simulink model "G24i_buck_boost"  (R2014a)
settings: Solver=ode23tb  StartTime=0.0  StopTime=5  RelTol=1e-4
values from neighbouring files (symbols this model uses):
  Array_Voc = [0.328644000009 2.76811 3.09396940822 3.26133568944 3.36629977409 3.44398192097 3.50365713438 3.55225637345 3.59363766529 3.63021764721 3.6624 3.69037314882 ... (101 elements, 101x1)]    [Array_Voc.mat]
  ArrayCurrent = [1.05303e-05 0.0329007487024 0.0659314357778 0.100205 0.132978217474 0.166891516648 0.200872978445 0.234107600227 0.267513340222 0.302009988541 0.336322 0.36979130469 ... (44440 elements, 101x440)]    [ArrayCurrent.mat]    (also in Genrate_SC_mod.m = fitresult_normal_g42(V,G); temp3.m = fitresult(V,G))
  ArrayVoltage = [0 0.01 0.02 0.03 0.04 0.05 0.06 0.07 0.08 0.09 0.1 0.11 ... (440 elements, 1x440)]    [ArrayVoltage.mat]    (also in Genrate_SC_mod.m = (0:0.01:max(Voltage)); temp3.m = (0:0.01:max(Voltage)))
  Irradiance = (min(Lux):50:max(Lux))    [Genrate_SC_mod.m]    (also in Irradiance.mat = [0 50 100 150 200 250 300 350 400 450 500 550 ... (101 eleme; temp3.m)
undefined symbols (not defined in the file or in its folder): sigbuilder_block
libraries: powerlib x16, simulink_extras x3, simulink x1
settings Model: NumberOfSteps=5  Creator=kartik.karuna  LastModifiedBy=kartik.karuna
settings SolverCC: SolverJacobianMethodControl=SparseAnalytical  ZeroCrossAlgorithm=Adaptive

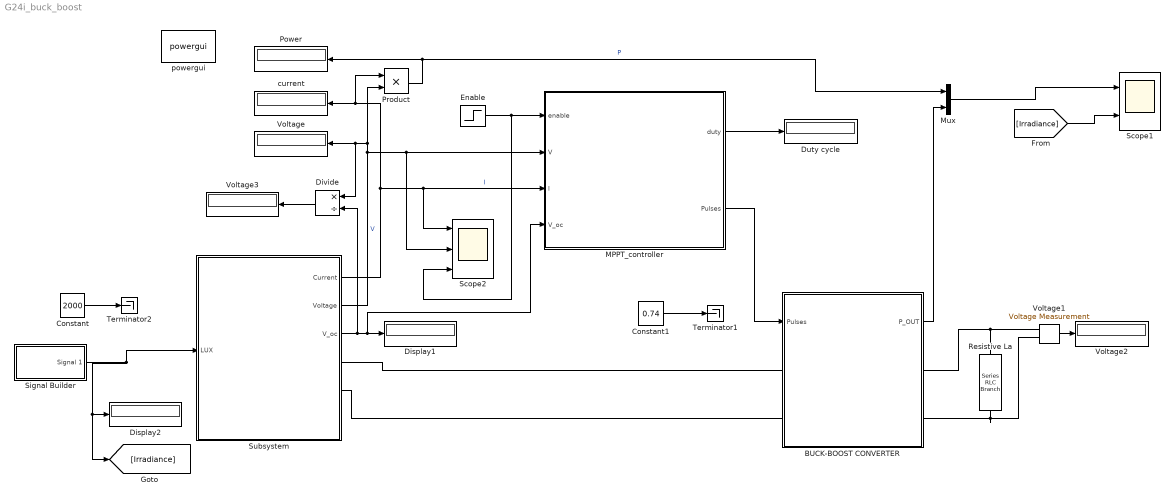
== system G24i_buck_boost ==
  BUCK-BOOST CONVERTER : Subsystem
  Constant : Constant  Value=2000
  Constant1 : Constant  Value=0.74
  Display1 : Display
  Display2 : Display
  Divide : Product  Inputs=*/
  Duty cycle : Display
  Enable : Step  Time=0.02  SampleTime=0
  MPPT_controller : Subsystem  Variant=on
  Mux : Mux  Inputs=2
  Power : Display
  Product : Product  RndMeth=Zero
  Resistive La : powerlib/Elements/Series RLC Branch  LConnTagsString=__new0  RConnTagsString=__new0  BranchType=R  Resistance=30  Inductance=1e-3  SetiL0=off  InitialCurrent=0  Capacitance=1e-6  Setx0=off  InitialVoltage=0  Measurements=None
  Scope1 : Scope  NumInputPorts=2
      settings: TimeRange=0.5  YMin=0~300  YMax=5.75~2500  SaveName=ScopeData2
  Scope2 : Scope  NumInputPorts=3
      settings: TimeRange=0.09  YMin=0.3125~3.9575~0.95  YMax=0.3475~3.968~1.05
  Signal Builder : Subsystem  Tag=STV Subsys  LoadFcn=sigbuilder_block('load');  StartFcn=sigbuilder_block('start');  StopFcn=sigbuilder_block('stop');  ClipboardFcn=sigbuilder_block('clipboard');  mask(Sigbuilder block){}
      mask help: Simulink:masks:SigbuilderBlock_MD
      mask init:
      | if ~strcmp(get_param(bdroot(gcbh),'SimulationStatus'),'stopped') tuvar = sigbuilder_block('maskInit'); end
      settings: CopyFcn=sigbuilder_block('copy');  DeleteFcn=sigbuilder_block('delete');  ModelCloseFcn=sigbuilder_block('modelClose');  PreSaveFcn=sigbuilder_block('preSave');  PauseFcn=sigbuilder_block('pause');  ContinueFcn=sigbuilder_block('continue');  NameChangeFcn=sigbuilder_block('namechange');  OpenFcn=sigbuilder_block('open',[310.966 125.379 1271.79 657.31 ]);  CloseFcn=sigbuilder_block('close');
      mask Display: plot(0, 0, 100, 100,[2, 2, 32, 32, 2], [68, 8, 8, 68, 68],[32, 2], [38, 38], [32, 19, 2],[53, 60, 44], [32, 17, 17, 2],[16, 16, 31, 31]);txt = getActiveGroup(gcbh);text(2, 100, txt,'verticalAlignment', 'top');
  Subsystem : Subsystem
  Terminator1 : Terminator
  Terminator2 : Terminator
  Voltage : Display
  Voltage1 : powerlib/Measurements/Voltage Measurement  PhasorSimulation=off  OutputType=Complex  PSBequivalent=0
  Voltage2 : Display
  Voltage3 : Display
  current : Display
  powergui : powerlib/powergui  Priority=1  SimulationMode=Continuous  SolverType=Tustin  SampleTime=50e-6  frequency=50  SPID=off  DisableSnubberDevices=off  DisableRonSwitches=off  DisableVfSwitches=off  SwTol=0  Interpol=off  DisplayEquations=off  Ts=0  methode=off  frequencyindice=0  Pbase=100e6  ErrMax=1e-4  Iterations=50  UnitsV=kV  UnitsW=MW  FunctionMessages=off  echomessages=off  HookPort=off  EnableUseOfTLC=off  x0status=blocks  RestoreLinks=warning  ResistiveCurrentMeasurement=off  Frange=[0:2:500]  Ylog=off  Xlog=on  ShowGrid=off  save=off  variable=ZData  structure=0  ZoomFFT=off  StartTime=0.0  cycles=1  DisplayStyle=1  fundamental=60  FreqAxis=off  MaxFrequency=1000  frequencyindicesteady=1  RmsSteady=1  display=off
  wires:
  BUCK-BOOST CONVERTER/1(P_OUT) -> Mux/2
  Mux/1 -> Scope1/1
  Product/1 -> Power/1, Mux/1  "P"
  Voltage1/1 -> Voltage2/1
  Enable/1 -> MPPT_controller/1(enable), Scope2/3
  Subsystem/3("V_oc ") -> Divide/2, MPPT_controller/4(V_oc), Display1/1
  Divide/1 -> Voltage3/1
  MPPT_controller/1(duty) -> Duty cycle/1
  Signal Builder/1(Signal 1) -> [Irradiance], Display2/1, Subsystem/1(LUX)
  Subsystem/2(Voltage) -> Product/2, Divide/1, Voltage/1, MPPT_controller/2(V), Scope2/2  "V"
  Subsystem/1(Current) -> Product/1, current/1, MPPT_controller/3(I), Scope2/1  "I"
  MPPT_controller/2(Pulses) -> BUCK-BOOST CONVERTER/1(Pulses)
  Constant1/1 -> Terminator1/1
  Constant/1 -> Terminator2/1
  [Irradiance] -> Scope1/2
  connections:
  Resistive La/RConn1 -- Voltage1/LConn2 -- BUCK-BOOST CONVERTER/RConn2
  Resistive La/LConn1 -- Voltage1/LConn1 -- BUCK-BOOST CONVERTER/RConn1
  BUCK-BOOST CONVERTER/LConn1 -- Subsystem/RConn1
  BUCK-BOOST CONVERTER/LConn2 -- Subsystem/RConn2

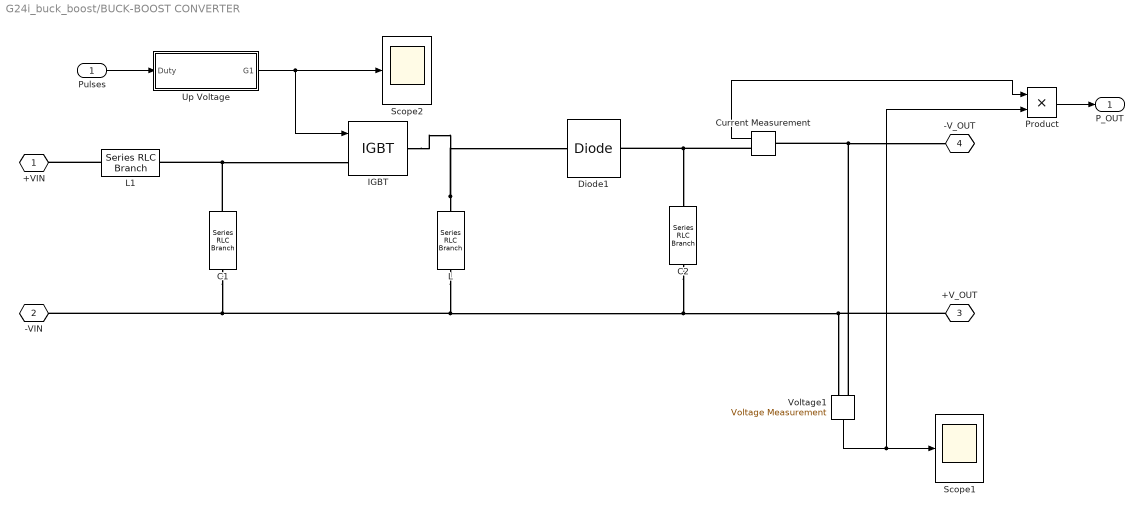
== system G24i_buck_boost/BUCK-BOOST CONVERTER ==
  Pulses : Inport
  " C1" : powerlib/Elements/Series RLC Branch  LConnTagsString=__new0  RConnTagsString=__new0  BranchType=C  Resistance=5  Inductance=0.05  SetiL0=off  InitialCurrent=0  Capacitance=2000e-6  Setx0=on  InitialVoltage=0  Measurements=Branch voltage and current
  " C2" : powerlib/Elements/Series RLC Branch  LConnTagsString=__new0  RConnTagsString=__new0  BranchType=C  Resistance=5  Inductance=0.05  SetiL0=off  InitialCurrent=0  Capacitance=2000e-6  Setx0=on  InitialVoltage=0  Measurements=Branch voltage and current
  " L" : powerlib/Elements/Series RLC Branch  LConnTagsString=__new0  RConnTagsString=__new0  BranchType=L  Resistance=5  Inductance=47e-6  SetiL0=on  InitialCurrent=0  Capacitance=1.0  Setx0=off  InitialVoltage=0  Measurements=Branch voltage and current
  " L1" : powerlib/Elements/Series RLC Branch  LConnTagsString=__new0  RConnTagsString=__new0  BranchType=L  Resistance=5  Inductance=1000e-6  SetiL0=on  InitialCurrent=0  Capacitance=1.0  Setx0=off  InitialVoltage=0  Measurements=Branch voltage and current
  Current Measurement : powerlib/Measurements/Current Measurement  PhasorSimulation=off  OutputType=Complex  PSBequivalent=0
  Diode1 : powerlib/Power Electronics/Diode  Ron=0.00001  Lon=0  Vf=0.8  IC=0  UseSnubber=off  Rs=1e4  Cs=1e-4  Measurements=off
  IGBT : powerlib/Power Electronics/IGBT  Ron=0.00001  Lon=0  Vf=2.5  Tf=1e-6  Tt=1e4  IC=0  Rs=1e5  Cs=inf  Measurements=off
  Product : Product  RndMeth=Zero
  Scope1 : Scope
      settings: TimeRange=1  YMin=1.478  YMax=1.497
  Scope2 : Scope
      settings: TimeRange=1  YMin=1.478  YMax=1.497  SaveName=ScopeData3
  Up Voltage : Subsystem  mask{fc=10000, Gama=0.5}
      mask prompts: fc "Frequency (Hz)"; Gama "Duty Cycle  (0-1)"
      mask Display: disp('CONTROL SIGNAL')
  Voltage1 : powerlib/Measurements/Voltage Measurement  PhasorSimulation=off  OutputType=Complex  PSBequivalent=0
  +VIN : PMIOPort  Tag=PMCPort  Port=1  Side=Left
  -VIN : PMIOPort  Tag=PMCPort  Port=2  Side=Left
  +V_OUT : PMIOPort  Tag=PMCPort  Port=3  Side=Right
  -V_OUT : PMIOPort  Tag=PMCPort  Port=4  Side=Right
  P_OUT : Outport
  wires:
  Voltage1/1 -> Scope1/1, Product/2
  Pulses/1 -> Up Voltage/1(Duty)
  Up Voltage/1(G1) -> IGBT/1, Scope2/1
  Current Measurement/1 -> Product/1
  Product/1 -> P_OUT/1
  connections:
  Voltage1/LConn2 -- -V_OUT/RConn1 -- Current Measurement/LConn1
  " L"/RConn1 -- +V_OUT/RConn1 -- Voltage1/LConn1 -- " C2"/RConn1 -- " C1"/RConn1 -- -VIN/RConn1
  " L"/LConn1 -- IGBT/RConn1 -- Diode1/RConn1
  " C1"/LConn1 -- IGBT/LConn1 -- " L1"/LConn1
  Current Measurement/RConn1 -- Diode1/LConn1 -- " C2"/LConn1
  " L1"/RConn1 -- +VIN/RConn1

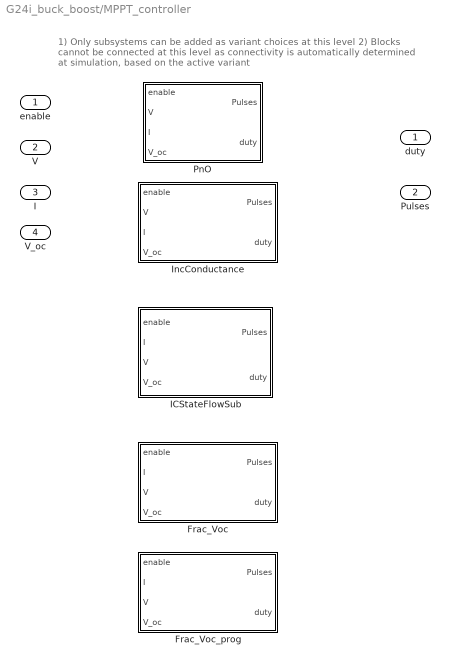
== system G24i_buck_boost/MPPT_controller ==
  note: 1) Only subsystems can be added as variant choices at this level
      | 2) Blocks cannot be connected at this level as connectivity is
      | automatically determined at simulation, based on the active variant
  enable : Inport
  V : Inport  Port=2
  I : Inport  Port=3
  V_oc : Inport  Port=4
  Frac_Voc : Subsystem  VariantControl=MPPT_Frac_Voc
  Frac_Voc_prog : Subsystem  VariantControl=MPPT_Frac_Voc_prog
  ICStateFlowSub : Subsystem  VariantControl=MPPT_IC_SF
  IncConductance : Subsystem  VariantControl=MPPT_IC_logic
  PnO : Subsystem  VariantControl=MPPT_PnO
  duty : Outport
  Pulses : Outport  Port=2

== system G24i_buck_boost/Signal Builder ==
  Demux : Demux  Tag=STV Demux  Outputs=1
  FromWs : FromWorkspace  Tag=STV FromWs  VariableName=tuvar  SampleTime=0
      SigBuilderData=|
      | common.afterFinalStr = 'Extrapolate'
      | common.sampleTime = 0
      | dataSet.timeRange = [0 2]
      | dataSet.name = 'Group 1'
      | sbobj.Groups.Name = 'Group 1'
      | sbobj.Groups.Signals.Name = 'Signal 1'
      | sbobj.Groups.Signals.XData = [0 0.35 0.55 0.85 1.2 2]
      | sbobj.Groups.Signals.YData = [2500 2500 200 200 800 800]
      | sbobj.Groups.TimeRange = [0 2]
  Signal 1 : Outport  Tag=STV Outport
  wires:
  Demux/1 -> Signal 1/1
  FromWs/1 -> Demux/1

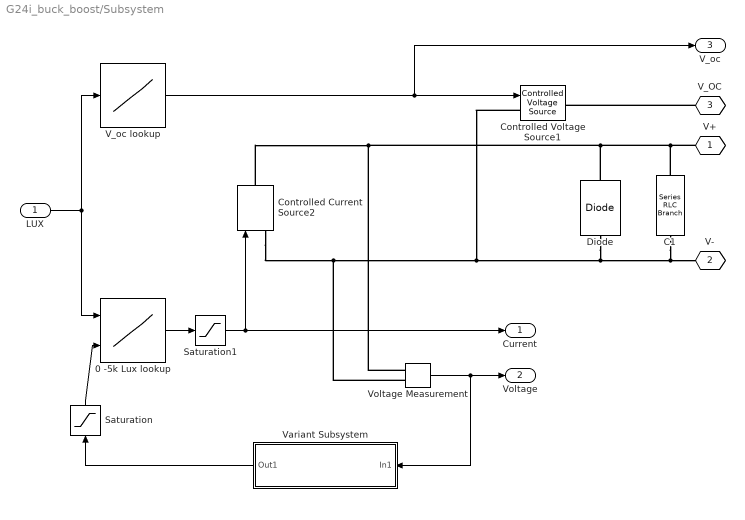
== system G24i_buck_boost/Subsystem ==
  LUX : Inport
  " C1" : powerlib/Elements/Series RLC Branch  LConnTagsString=__new0  RConnTagsString=__new0  BranchType=C  Resistance=5  Inductance=0.05  SetiL0=off  InitialCurrent=0  Capacitance=100e-6  Setx0=on  InitialVoltage=0  Measurements=Branch voltage and current
  0 -5k Lux lookup : Lookup_n-D  BreakpointsForDimension1=Irradiance  BreakpointsForDimension2=ArrayVoltage  BreakpointsForDimension1Min=[0]  BreakpointsForDimension2Min=[0]  BreakpointsForDimension1Max=[5000]  BreakpointsForDimension2Max=[6]  Table=ArrayCurrent  DiagnosticForOutOfRangeInput=Warning  RndMeth=Simplest  InputSameDT=on
  Controlled Current Source2 : powerlib/Electrical Sources/Controlled Current Source  Initialize=on  Source_Type=DC  Amplitude=0  Phase=0  Frequency=0  Measurements=None
  Controlled Voltage Source1 : powerlib/Electrical Sources/Controlled Voltage Source  Initialize=on  Source_Type=AC  Amplitude=0  Phase=0  Frequency=0  Measurements=Voltage
  Diode : powerlib/Power Electronics/Diode  Ron=0.001  Lon=0  Vf=0  IC=0  UseSnubber=off  Rs=500  Cs=250e-9  Measurements=off
  Saturation : Saturate  UpperLimit=6  LowerLimit=0
  Saturation1 : Saturate  UpperLimit=6  LowerLimit=-1
  V_oc lookup : Lookup_n-D  NumberOfTableDimensions=1  BreakpointsForDimension1=Irradiance  Table=Array_Voc  RndMeth=Simplest  InputSameDT=on
  Variant Subsystem : Subsystem  Variant=on
  Voltage Measurement : powerlib/Measurements/Voltage Measurement  PhasorSimulation=off  OutputType=Complex  PSBequivalent=0
  V+ : PMIOPort  Tag=PMCPort  Port=1  Side=Right
  V- : PMIOPort  Tag=PMCPort  Port=2  Side=Right
  V_OC : PMIOPort  Tag=PMCPort  Port=3  Side=Right
  Current : Outport
  Voltage : Outport  Port=2
  "V_oc " : Outport  Port=3
  wires:
  LUX/1 -> 0 -5k Lux lookup/1, V_oc lookup/1
  Voltage Measurement/1 -> Variant Subsystem/1(In1), Voltage/1
  Variant Subsystem/1(Out1) -> Saturation/1
  0 -5k Lux lookup/1 -> Saturation1/1
  V_oc lookup/1 -> "V_oc "/1, Controlled Voltage Source1/1
  Saturation/1 -> 0 -5k Lux lookup/2
  Saturation1/1 -> Controlled Current Source2/1, Current/1
  connections:
  Controlled Current Source2/RConn1 -- V+/RConn1 -- " C1"/LConn1 -- Diode/RConn1 -- Voltage Measurement/LConn1
  Controlled Voltage Source1/LConn1 -- Voltage Measurement/LConn2 -- Controlled Current Source2/LConn1 -- Diode/LConn1 -- V-/RConn1 -- " C1"/RConn1
  V_OC/RConn1 -- Controlled Voltage Source1/RConn1

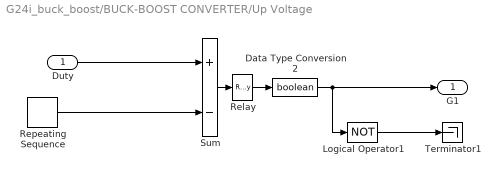
== system G24i_buck_boost/BUCK-BOOST CONVERTER/Up Voltage ==
  Duty : Inport
  Data Type Conversion2 : DataTypeConversion  OutDataTypeStr=boolean  SaturateOnIntegerOverflow=on  RndMeth=Zero
  Logical Operator1 : Logic  Operator=NOT
  Relay : Relay  ZeroCross=off
  Repeating Sequence : simulink/Sources/Repeating Sequence  rep_seq_t=[0 1/10e3]  rep_seq_y=[0 1]
  Sum : Sum  Inputs=+-  SaturateOnIntegerOverflow=on  InputSameDT=on  OutDataTypeStr=Inherit: Same as first input
  Terminator1 : Terminator
  G1 : Outport
  wires:
  Data Type Conversion2/1 -> Logical Operator1/1, G1/1
  Duty/1 -> Sum/1
  Repeating Sequence/1 -> Sum/2
  Sum/1 -> Relay/1
  Relay/1 -> Data Type Conversion2/1
  Logical Operator1/1 -> Terminator1/1

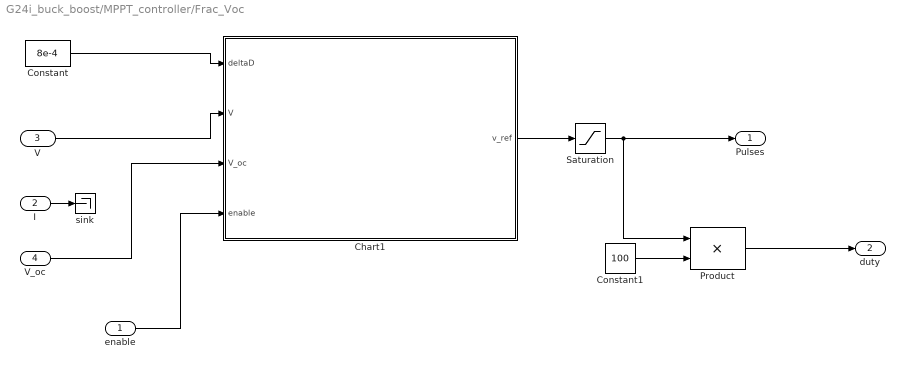
== system G24i_buck_boost/MPPT_controller/Frac_Voc ==
  enable : Inport
  I : Inport  Port=2
  V : Inport  Port=3
  V_oc : Inport  Port=4
  Chart1 : Stateflow chart  TreatAsAtomicUnit=on
  Constant : Constant  Value=8e-4
  Constant1 : Constant  Value=100
  Product : Product  RndMeth=Zero
  Saturation : Saturate  UpperLimit=.95  LowerLimit=0.1
  sink : Terminator
  Pulses : Outport
  duty : Outport  Port=2
  wires:
  Constant/1 -> Chart1/1(deltaD)
  V/1 -> Chart1/2(V)
  enable/1 -> Chart1/4(enable)
  Chart1/1(v_ref) -> Saturation/1
  Saturation/1 -> Pulses/1, Product/1
  Constant1/1 -> Product/2
  Product/1 -> duty/1
  V_oc/1 -> Chart1/3(V_oc)
  I/1 -> sink/1

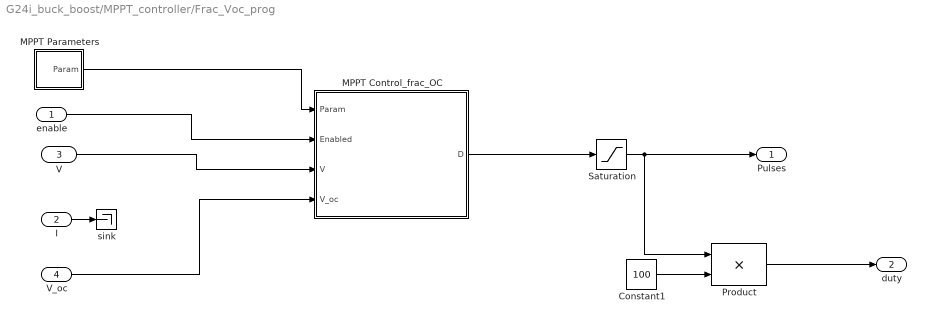
== system G24i_buck_boost/MPPT_controller/Frac_Voc_prog ==
  enable : Inport
  I : Inport  Port=2
  V : Inport  Port=3
  V_oc : Inport  Port=4
  Constant1 : Constant  Value=100
  MPPT Parameters : Subsystem
  "MPPT Control_frac_OC " : MATLAB Function  TreatAsAtomicUnit=on
  Product : Product  RndMeth=Zero
  Saturation : Saturate  UpperLimit=.95  LowerLimit=0.1
  sink : Terminator
  Pulses : Outport
  duty : Outport  Port=2
  wires:
  MPPT Parameters/1(Param) -> "MPPT Control_frac_OC "/1(Param)
  V/1 -> "MPPT Control_frac_OC "/3(V)
  enable/1 -> "MPPT Control_frac_OC "/2(Enabled)
  "MPPT Control_frac_OC "/1(D) -> Saturation/1
  Saturation/1 -> Pulses/1, Product/1
  Constant1/1 -> Product/2
  Product/1 -> duty/1
  V_oc/1 -> "MPPT Control_frac_OC "/4(V_oc)
  I/1 -> sink/1

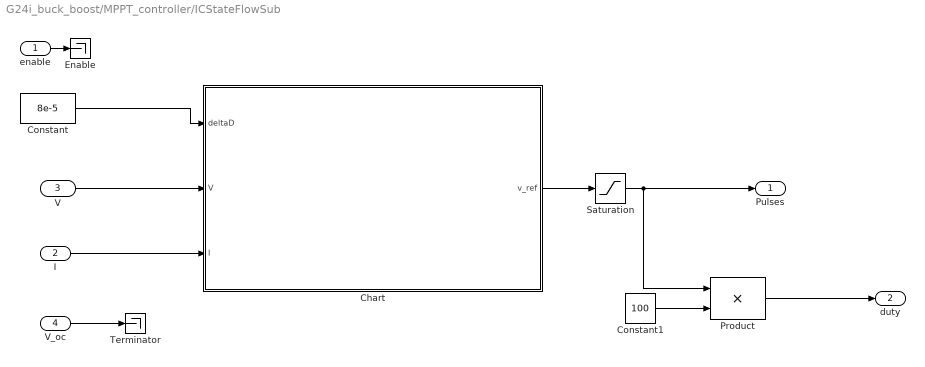
== system G24i_buck_boost/MPPT_controller/ICStateFlowSub ==
  enable : Inport
  I : Inport  Port=2
  V : Inport  Port=3
  V_oc : Inport  Port=4
  Chart : Stateflow chart  TreatAsAtomicUnit=on
  Constant : Constant  Value=8e-5
  Constant1 : Constant  Value=100
  "Enable " : Terminator
  Product : Product  RndMeth=Zero
  Saturation : Saturate  UpperLimit=.95  LowerLimit=0.1
  Terminator : Terminator
  Pulses : Outport
  duty : Outport  Port=2
  wires:
  I/1 -> Chart/3(I)
  Constant/1 -> Chart/1(deltaD)
  V/1 -> Chart/2(V)
  enable/1 -> "Enable "/1
  Chart/1(v_ref) -> Saturation/1
  Saturation/1 -> Pulses/1, Product/1
  Constant1/1 -> Product/2
  Product/1 -> duty/1
  V_oc/1 -> Terminator/1

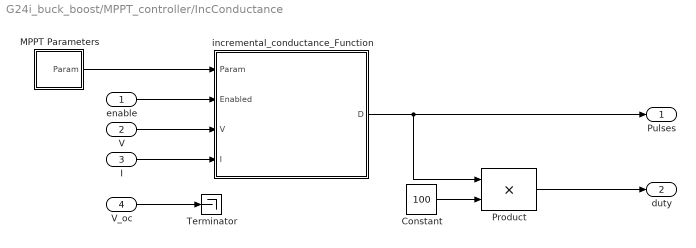
== system G24i_buck_boost/MPPT_controller/IncConductance ==
  enable : Inport
  V : Inport  Port=2
  I : Inport  Port=3
  V_oc : Inport  Port=4
  Constant : Constant  Value=100
  MPPT Parameters : Subsystem
  Product : Product  RndMeth=Zero
  Terminator : Terminator
  "incremental_conductance_Function " : MATLAB Function  TreatAsAtomicUnit=on
  Pulses : Outport
  duty : Outport  Port=2
  wires:
  V/1 -> "incremental_conductance_Function "/3(V)
  I/1 -> "incremental_conductance_Function "/4(I)
  Constant/1 -> Product/2
  Product/1 -> duty/1
  "incremental_conductance_Function "/1(D) -> Pulses/1, Product/1
  enable/1 -> "incremental_conductance_Function "/2(Enabled)
  V_oc/1 -> Terminator/1
  MPPT Parameters/1(Param) -> "incremental_conductance_Function "/1(Param)

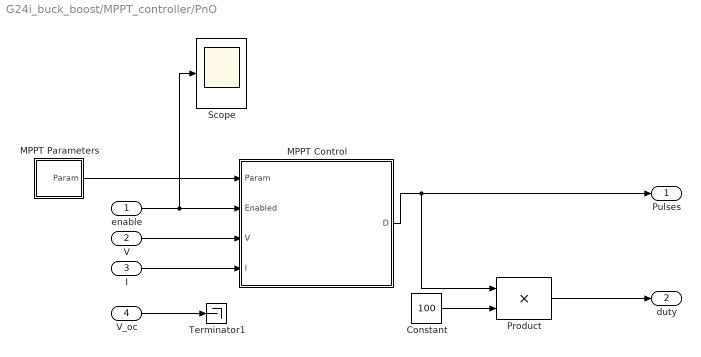
== system G24i_buck_boost/MPPT_controller/PnO ==
  enable : Inport
  V : Inport  Port=2
  I : Inport  Port=3
  V_oc : Inport  Port=4
  Constant : Constant  Value=100
  MPPT Parameters : Subsystem
  "MPPT Control " : MATLAB Function  TreatAsAtomicUnit=on
  Product : Product  RndMeth=Zero
  Scope : Scope
      settings: TimeRange=1  YMin=-4.16334e-17  YMax=0.6  SaveName=ScopeData4
  Terminator1 : Terminator
  Pulses : Outport
  duty : Outport  Port=2
  wires:
  enable/1 -> "MPPT Control "/2(Enabled), Scope/1
  V_oc/1 -> Terminator1/1
  MPPT Parameters/1(Param) -> "MPPT Control "/1(Param)
  V/1 -> "MPPT Control "/3(V)
  I/1 -> "MPPT Control "/4(I)
  "MPPT Control "/1(D) -> Pulses/1, Product/1
  Constant/1 -> Product/2
  Product/1 -> duty/1

== system G24i_buck_boost/Subsystem/Variant Subsystem ==
  note: 1) Only subsystems can be added as variant choices at this level
      | 2) Blocks cannot be connected at this level as connectivity is
      | automatically determined at simulation, based on the active variant
  In1 : Inport
  Transfer Fcn Default : simulink_extras/Additional Linear/Transfer Fcn (with initial states)  VariantControl=(default)  N=[1]  D="[.01  1]"  X0=0
  Transfer Fcn PnO : simulink_extras/Additional Linear/Transfer Fcn (with initial states)  VariantControl=MPPT_PnO  N=[1]  D="[.0001  1]"  X0=0
  Transfer Fcn1 inC : simulink_extras/Additional Linear/Transfer Fcn (with initial states)  VariantControl=MPPT_IC_logic  N=[1]  D="[.001  1]"  X0=0
  Out1 : Outport

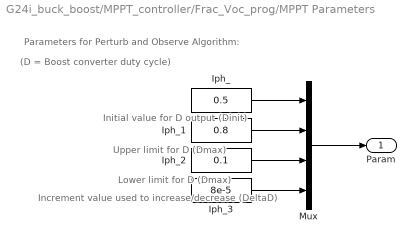
== system G24i_buck_boost/MPPT_controller/Frac_Voc_prog/MPPT Parameters ==
  note: Upper limit for D (Dmax)
  note: Increment value used to increase/decrease (DeltaD)
  note: Initial value for D output (Dinit)
  note: (D = Boost converter duty cycle)
  note: Lower limit for D (Dmax)
  note: Parameters for Perturb and Observe Algorithm:
  Iph_ : Constant  Value=0.5
  Iph_1 : Constant  Value=0.8
  Iph_2 : Constant  Value=0.1
  Iph_3 : Constant  Value=8e-5
  Mux : Mux
  Param : Outport
  wires:
  Iph_/1 -> Mux/1
  Iph_1/1 -> Mux/2
  Iph_2/1 -> Mux/3
  Iph_3/1 -> Mux/4
  Mux/1 -> Param/1

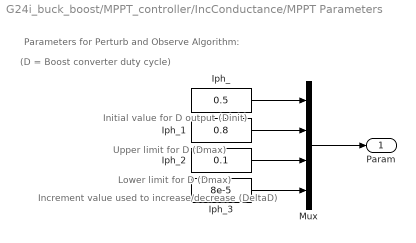
== system G24i_buck_boost/MPPT_controller/IncConductance/MPPT Parameters ==
  note: Upper limit for D (Dmax)
  note: Increment value used to increase/decrease (DeltaD)
  note: Initial value for D output (Dinit)
  note: (D = Boost converter duty cycle)
  note: Lower limit for D (Dmax)
  note: Parameters for Perturb and Observe Algorithm:
  Iph_ : Constant  Value=0.5
  Iph_1 : Constant  Value=0.8
  Iph_2 : Constant  Value=0.1
  Iph_3 : Constant  Value=8e-5
  Mux : Mux
  Param : Outport
  wires:
  Iph_/1 -> Mux/1
  Iph_1/1 -> Mux/2
  Iph_2/1 -> Mux/3
  Iph_3/1 -> Mux/4
  Mux/1 -> Param/1

== system G24i_buck_boost/MPPT_controller/PnO/MPPT Parameters ==
  note: Upper limit for D (Dmax)
  note: Increment value used to increase/decrease (DeltaD)
  note: Initial value for D output (Dinit)
  note: (D = Boost converter duty cycle)
  note: Lower limit for D (Dmax)
  note: Parameters for Perturb and Observe Algorithm:
  Iph_ : Constant  Value=0.5
  Iph_1 : Constant  Value=0.95
  Iph_2 : Constant  Value=0.1
  Iph_3 : Constant  Value=15e-5
  Mux : Mux
  Param : Outport
  wires:
  Iph_/1 -> Mux/1
  Iph_1/1 -> Mux/2
  Iph_2/1 -> Mux/3
  Iph_3/1 -> Mux/4
  Mux/1 -> Param/1

== matlab function G24i_buck_boost/MPPT_controller/IncConductance/incremental_conductance_Function  ==
  settings: updateMethod=DISCRETE  sampleTime=Ts_Control
  data: Param input; Enabled input; V input; I input; D output
function D  = IncC_Pog(Param, Enabled, V, I)
% MPPT controller block based on the incremental conductance algorithm
% MPPT controller based on the Perturb & Observe algorithm.

% D output = Duty cycle  (value between 0 and 1)
%
% Enabled input = 1 to enable the MPPT controller
% V input = PV array terminal voltage (V)
% I input = PV array current (A)
%
% Param input:
Dinit = Param(1);  %Initial value for D output
Dmax = Param(2);   %Maximum value for D
Dmin = Param(3);   %Minimum value for D
deltaD = Param(4); %Increment value used to increase/decrease the duty cycle D

% ( increasing D = decreasing Vref )
persistent Vold Dold Iold;

dataType = 'double';

if isempty(Vold)
    Vold=0;
    Iold=0;
    Dold=Dinit;
    D=Dinit;
    
end

dV= V - Vold;
dI= I- Iold;


if Enabled == 1
   if dV==0
       if dI ~= 0
           if dI >0
               D = Dold + deltaD;
           else 
               D = Dold + deltaD;
           end
       else
           D=Dold;
       end
       Dold=D;
       Vold=V;
       Iold=I;
   else
       if ((dI/dV) ~= (-I/V))
           if ((dI/dV) > (-I/V))
               D = Dold - deltaD;
           else 
               D = Dold + deltaD;
           end
       else
           D=Dold;
       end
       Dold=D;
       Vold=V;
       Iold=I;
   end
  
else
    D=Dold;
end

if D >= Dmax | D<= Dmin
    D=Dold;
end

== matlab function G24i_buck_boost/MPPT_controller/Frac_Voc_prog/MPPT Control_frac_OC  ==
  settings: updateMethod=DISCRETE  sampleTime=Ts_Control
  data: Param input; Enabled input; V input; V_oc input; D output
function D  = frac_oc(Param, Enabled, V, V_oc)

% MPPT controller based on the Perturb & Observe algorithm.

% D output = Duty cycle  (value between 0 and 1)
%
% Enabled input = 1 to enable the MPPT controller
% V input = PV array terminal voltage (V)
% I input = PV array current (A)
%
% Param input:
Dinit = Param(1);  %Initial value for D output
Dmax = Param(2);   %Maximum value for D
Dmin = Param(3);   %Minimum value for D
deltaD = Param(4); %Increment value used to increase/decrease the duty cycle D
% ( increasing D = decreasing Vref )


persistent  Dold;

dataType = 'double';

if isempty(Dold)
      Dold=Dinit;
end
Vmpp = ((0.9501)*V_oc)-0.4825; 
dV= V - Vmpp;


if dV ~= 0 && Enabled ~=0
    
        if dV > 0
            D = Dold + deltaD;
        else
            D = Dold - deltaD;
        end
   
   
else D=Dold;
end

if D >= Dmax || D<= Dmin
    D=Dold;
end

Dold=D;

== stateflow chart G24i_buck_boost/MPPT_controller/ICStateFlowSub/Chart ==
  state init
    entry:
    V_prev1=0;
    I_prev1=0;
    V_REF=0.5;
  state Sample_and_call
    entry:
    deltaV = V -V_prev1;
    deltaI = I - I_prev1;
    v_ref = V_REF;
  state INCREMENT
    entry:
    v_ref =v_ref+deltaD;
  state DECREMENT
    entry:
    v_ref =v_ref-deltaD;
  state RETURN
    entry:
    V_prev1 = V;
    I_prev1 = I ;
    V_REF= v_ref;
  (default) -> init
  init -> Sample_and_call
  RETURN -> Sample_and_call
  Sample_and_call -> (junction 35)
  (junction 35) -> (junction 6) [order 2] : [deltaV==0]
  (junction 35) -> (junction 22) [order 1] : [deltaV~=0]
  (junction 6) -> RETURN [order 2] : [deltaI==0]
  (junction 6) -> (junction 16) [order 1] : [deltaI~=0]
  (junction 22) -> RETURN [order 2] : [deltaI/deltaV == -(I/V)]
  (junction 22) -> (junction 15) [order 1] : [deltaI/deltaV ~= -(I/V)]
  (junction 16) -> DECREMENT [order 2] : [deltaI<=0]
  (junction 16) -> INCREMENT [order 1] : [deltaI>0]
  (junction 15) -> INCREMENT [order 2]
  (junction 15) -> DECREMENT [order 1] : [(deltaI/deltaV) > -(I/V)]
  INCREMENT -> RETURN
  DECREMENT -> RETURN
  data: deltaD input; v_ref output double; V_prev1 local =0; I_prev1 local =0; V_REF local =0; deltaV local; deltaI local; V input; I input

== matlab function G24i_buck_boost/MPPT_controller/PnO/MPPT Control  ==
  settings: updateMethod=DISCRETE  sampleTime=Ts_Control
  data: Param input; Enabled input; V input; I input; D output
function D  = PandO(Param, Enabled, V, I)

% MPPT controller based on the Perturb & Observe algorithm.

% D output = Duty cycle  (value between 0 and 1)
%
% Enabled input = 1 to enable the MPPT controller
% V input = PV array terminal voltage (V)
% I input = PV array current (A)
%
% Param input:
Dinit = Param(1);  %Initial value for D output
Dmax = Param(2);   %Maximum value for D
Dmin = Param(3);   %Minimum value for D
deltaD = Param(4); %Increment value used to increase/decrease the duty cycle D
% ( increasing D = decreasing Vref )


persistent Vold Pold Dold;

dataType = 'double';

if isempty(Vold)
    Vold=0;
    Pold=0;
    Dold=Dinit;
end
P= V*I;
dV= V - Vold;
dP= P - Pold;

if dP ~= 0 & Enabled ~=0
    if dP < 0
        if dV < 0
            D = Dold - deltaD;
        else
            D = Dold + deltaD;
        end
    else
        if dV < 0
            D = Dold + deltaD;
        else
            D = Dold - deltaD;
        end    
    end
else D=Dold;
end

if D >= Dmax | D<= Dmin
    D=Dold;
end

Dold=D;
Vold=V;
Pold=P;

== stateflow chart G24i_buck_boost/MPPT_controller/Frac_Voc/Chart1 ==
  state init
    entry:
    V_REF=0.5;
    Vmpp=(0.9501)*(V_oc)-(0.4825);
  state Sample_and_call
    entry:
    deltaV = V -Vmpp;
    v_ref = V_REF;
  state INCREMENT
    entry:
    v_ref =v_ref+deltaD;
  state DECREMENT
    entry:
    v_ref =v_ref-deltaD;
  state RETURN
    entry:
    V_REF= v_ref;
  (default) -> init
  init -> Sample_and_call
  RETURN -> Sample_and_call
  Sample_and_call -> (junction 15)
  (junction 15) -> RETURN [order 2] : [deltaV==0]
  (junction 15) -> (junction 5) [order 1] : [deltaV~=0]
  (junction 5) -> DECREMENT [order 2] : [deltaV>0]
  (junction 5) -> INCREMENT [order 1] : [deltaV<0]
  INCREMENT -> RETURN
  DECREMENT -> RETURN
  data: deltaD input; Vmpp local; deltaV local; v_ref output; V_REF local; V input; V_oc input; enable input
